simulink model "comparando_modelos_mecanicos"  (R2012b)
settings: Solver=ode45  StartTime=0.0  StopTime=0.5  RelTol=1e-3
undefined symbols (not defined in the file): DF, DiscIntNeverNeededParam, J, Kd, P, Ts
libraries: simulink x2
settings Model: Creator=Juliano  LastModifiedBy=Juliano

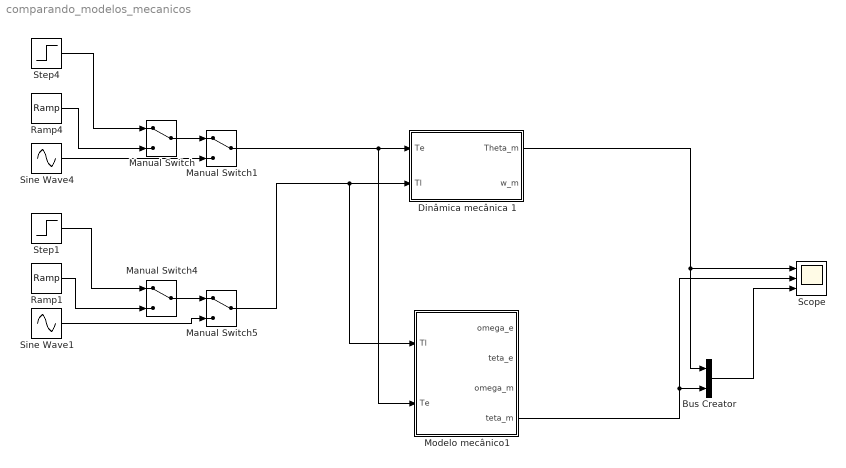
== system comparando_modelos_mecanicos ==
  Bus Creator : BusCreator  Inputs=2
  Dinâmica mecânica 1 : Subsystem
  Manual Switch{,1,4..5} (4 alike) : ManualSwitch
  Modelo mecânico1 : Subsystem
  Ramp1 : simulink/Sources/Ramp  slope=20  start=0  X0=0
  Ramp4 : simulink/Sources/Ramp  slope=2*pi  start=0  X0=0
  Scope : Scope  NumInputPorts=3
      settings: TimeRange=0.5  YMin=0~0~0  YMax=30000~30000~30000
  Sine Wave1 : Sin  SampleTime=0
  Sine Wave4 : Sin  SampleTime=0
  Step1 : Step  Time=0.2  After=10  SampleTime=0
  Step4 : Step  Time=0  After=5  SampleTime=0
  wires:
  Manual Switch/1 -> Manual Switch1/1
  Manual Switch4/1 -> Manual Switch5/1
  Step4/1 -> Manual Switch/1
  Ramp4/1 -> Manual Switch/2
  Sine Wave4/1 -> Manual Switch1/2
  Manual Switch5/1 -> Modelo mecânico1/1(Tl), Dinâmica mecânica 1/2(Tl)
  Bus Creator/1 -> Scope/3
  Manual Switch1/1 -> Modelo mecânico1/2(Te), Dinâmica mecânica 1/1(Te)
  Step1/1 -> Manual Switch4/1
  Ramp1/1 -> Manual Switch4/2
  Sine Wave1/1 -> Manual Switch5/2
  Dinâmica mecânica 1/1(Theta_m) -> Bus Creator/1, Scope/1
  Modelo mecânico1/4(teta_m) -> Scope/2, Bus Creator/2

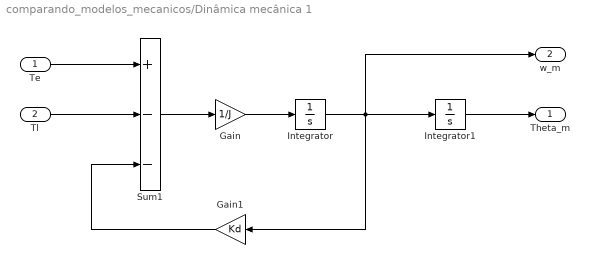
== system comparando_modelos_mecanicos/Dinâmica mecânica 1 ==
  Te : Inport
  Tl : Inport  Port=2
  Gain : Gain  Gain=1/J
  Gain1 : Gain  Gain=Kd
  Integrator : Integrator
  Integrator1 : Integrator
  Sum1 : Sum  Inputs=+--
  Theta_m : Outport
  w_m : Outport  Port=2
  wires:
  Sum1/1 -> Gain/1
  Gain/1 -> Integrator/1
  Integrator/1 -> w_m/1, Integrator1/1, Gain1/1
  Te/1 -> Sum1/1
  Gain1/1 -> Sum1/3
  Tl/1 -> Sum1/2
  Integrator1/1 -> Theta_m/1

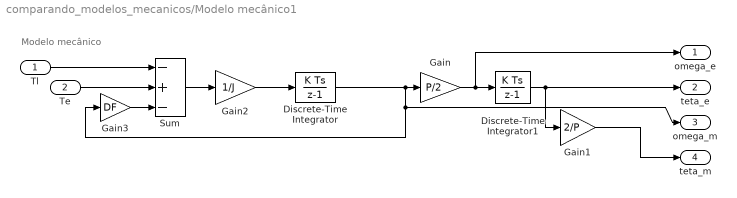
== system comparando_modelos_mecanicos/Modelo mecânico1 ==
  note: Modelo mecânico
  Tl : Inport
  Te : Inport  Port=2
  Discrete-Time Integrator : DiscreteIntegrator  SampleTime=Ts  ICPrevOutput=DiscIntNeverNeededParam  ICPrevScaledInput=DiscIntNeverNeededParam
  Discrete-Time Integrator1 : DiscreteIntegrator  SampleTime=Ts  ICPrevOutput=DiscIntNeverNeededParam  ICPrevScaledInput=DiscIntNeverNeededParam
  Gain : Gain  Gain=P/2  SaturateOnIntegerOverflow=on  OutDataTypeStr=Inherit: Same as input  ParamDataTypeStr=Inherit: Same as input
  Gain1 : Gain  Gain=2/P  SaturateOnIntegerOverflow=on  OutDataTypeStr=Inherit: Same as input  ParamDataTypeStr=Inherit: Same as input
  Gain2 : Gain  Gain=1/J  SaturateOnIntegerOverflow=on  OutDataTypeStr=Inherit: Same as input  ParamDataTypeStr=Inherit: Same as input
  Gain3 : Gain  Gain=DF  SaturateOnIntegerOverflow=on  OutDataTypeStr=Inherit: Same as input  ParamDataTypeStr=Inherit: Same as input
  Sum : Sum  Inputs=-+-  SaturateOnIntegerOverflow=on  InputSameDT=on  OutDataTypeStr=Inherit: Same as first input
  omega_e : Outport
  teta_e : Outport  Port=2
  omega_m : Outport  Port=3
  teta_m : Outport  Port=4
  wires:
  Gain1/1 -> teta_m/1
  Te/1 -> Sum/2
  Gain3/1 -> Sum/3
  Tl/1 -> Sum/1
  Sum/1 -> Gain2/1
  Gain2/1 -> Discrete-Time Integrator/1
  Discrete-Time Integrator/1 -> Gain/1, omega_m/1, Gain3/1
  Gain/1 -> omega_e/1, Discrete-Time Integrator1/1
  Discrete-Time Integrator1/1 -> Gain1/1, teta_e/1
